simulink library "NCS_Library"  (R2019a)
settings: Solver=VariableStepAuto  StartTime=0.0  StopTime=10.0  RelTol=1e-3
values from neighbouring files (symbols this model uses):
  A = 10    [Parameter.m]
  band = 100000000    [Parameter.m]
  BER = 0    [Parameter.m]
  c = 5000000    [Parameter.m]
  c1 = 4.33    [Parameter.m]
  c2 = 3.16    [Parameter.m]
  CAN2EthernetDelay = 0.000    (= 0)    [Parameter.m]
  cR = 1.5*10^-3    (= 0.0015)    [Parameter.m]
  cw = (cwE * 2 + cwM * (nW_ges-2))/nW_ges    (= 0.1475)    [Parameter.m]
  cwE = 0.35    [Parameter.m]
  cwM = 0.08    [Parameter.m]
  Cycle_Controller = 0    [Parameter.m]
  CyclePLC = 24/1000    (= 0.024)    [Parameter.m]
  d = 800000    [Parameter.m]
  Dr = 0.92    [Parameter.m]
  Ethernet2CANDelay = 0.005    [Parameter.m]
  F_konst = 70892    [Parameter.m]
  FA = 100000    [Parameter.m]
  FB_WB_max = 10000    [Parameter.m]
  FBel_an = iG*nG*F_KZmax*nBan*R_mR/(Dr/2)    (= 28197.4297239)    [Parameter.m]
  FBel_frei = iG*nG*F_KZmax*nBfrei*R_mW/(Dr/2)    (= 29270.6882948)    [Parameter.m]
  Fmaxdyn = 300000    [Parameter.m]
  g = 9.81    [Parameter.m]
  i = 0    [Parameter.m]
  J = 1/2*mA*(Dr/2)^2    (= 158.7)    [Parameter.m]
  k1 = 0.095    [Parameter.m]
  k2 = 9.26/3.6    (= 2.57222222222)    [Parameter.m]
  k3 = 4.63/3.6    (= 1.28611111111)    [Parameter.m]
  mges = 58000    [Parameter.m]
  mu = [mu1 mu2]    [Parameter.m]
  muBel1 = 0.42    [Parameter.m]
  muBel2 = 0.36    [Parameter.m]
  n = 0.001    [Parameter.m]
  n_Mg = 4    [Parameter.m]
  n_WB = 4    [Parameter.m]
  nA = 4    [Parameter.m]
  nBan = 2    [Parameter.m]
  nBfrei = 3    [Parameter.m]
  nM = 4    [Parameter.m]
  nW_an = 4    [Parameter.m]
  P_max = 8200000    [Parameter.m]
  Q = 10    [Parameter.m]
  r_reib = 600    [Parameter.m]
  rho = 1.08    [Parameter.m]
  rhoL = 1.225    [Parameter.m]
  Size = 8    [Parameter.m]
  slip = [s1 s2]    [Parameter.m]
  tol = 0.05    [Parameter.m]
  v00 = 100/3.6    (= 27.7777777778)    [Parameter.m]
  v_grenz = 60/3.6    (= 16.6666666667)    [Parameter.m]
  v_opt = 75/3.6    (= 20.8333333333)    [Parameter.m]
  W_opt = 0.5    [Parameter.m]
  WB = 1    [Parameter.m]
  y_opt = sqrt(W_opt)/((1+sqrt(W_opt))^2+W_opt)    [Parameter.m]
undefined symbols (not defined in the file or in its folder): BUSCapacity, CableLength, controlGate, D_dyn, D_mg, EnableBurst, EnableToF, entity, Entity_out, Gate, Gate_4, Gate_5, Gate_ACK, Gate_copy, Gate_RX, getData, gettime, I_dyn, I_mg, m, magnitude, P_dyn, P_mg, ReadAttributes, readdata, ReadData, ReadSize, sigbuilder_block, Timeout, ToB, ToF, v0, v_d, v_soll
libraries: simulink x176, $bdroot x102
(part 7 of 12)

== system NCS_Library/Network/ETB/Subsystem2/MAC Layer ==
  InIP1 : Inport
  InFromIP2 : Inport  Port=2
  InFromIP3 : Inport  Port=3
  Parameter : Inport  Port=4
  InFromSubnet1 : Inport  Port=5
  InFromSubnet2 : Inport  Port=6
  InFromSubnet3 : Inport  Port=7
  Failure Control{,1..11} (12 alike) : $bdroot/Network/Applications/Failure Control  SystemSampleTime=-1
  MAC Controller1 : $bdroot/Network/ETB/OSI Layers/MAC Controller  SystemSampleTime=-1
  MAC Controller2 : $bdroot/Network/ETB/OSI Layers/MAC Controller  SystemSampleTime=-1
  MAC Controller3 : $bdroot/Network/ETB/OSI Layers/MAC Controller  SystemSampleTime=-1
  Terminator{,1..5} (6 alike) : Terminator
  OutIP1 : Outport
  OutToIP2 : Outport  Port=2
  OutToIP3 : Outport  Port=3
  OutToSubnet1 : Outport  Port=4
  OutSubnet2 : Outport  Port=5
  OutToSubnet3 : Outport  Port=6
  wires:
  MAC Controller1/1 -> Failure Control9/1
  MAC Controller1/4 -> Failure Control8/1
  InFromIP2/1 -> Failure Control7/1
  InFromSubnet2/1 -> Failure Control6/1
  MAC Controller2/4 -> Failure Control4/1
  MAC Controller2/1 -> Failure Control5/1
  InFromIP3/1 -> Failure Control1/1
  MAC Controller3/1 -> Failure Control3/1
  MAC Controller3/4 -> Failure Control2/1
  InFromSubnet3/1 -> Failure Control/1
  Parameter/1 -> MAC Controller3/2, MAC Controller2/2, MAC Controller1/2
  MAC Controller2/2 -> Terminator/1
  MAC Controller2/3 -> Terminator1/1
  MAC Controller3/2 -> Terminator2/1
  MAC Controller3/3 -> Terminator3/1
  MAC Controller1/3 -> Terminator4/1
  MAC Controller1/2 -> Terminator5/1
  InIP1/1 -> Failure Control11/1
  InFromSubnet1/1 -> Failure Control10/1
  Failure Control/1 -> MAC Controller3/3
  Failure Control1/1 -> MAC Controller3/1
  Failure Control2/1 -> OutToSubnet3/1
  Failure Control3/1 -> OutToIP3/1
  Failure Control4/1 -> OutSubnet2/1
  Failure Control5/1 -> OutToIP2/1
  Failure Control6/1 -> MAC Controller2/3
  Failure Control7/1 -> MAC Controller2/1
  Failure Control8/1 -> OutToSubnet1/1
  Failure Control9/1 -> OutIP1/1
  Failure Control10/1 -> MAC Controller1/3
  Failure Control11/1 -> MAC Controller1/1

== system NCS_Library/Network/ETB/Subsystem2/Routing Layer ==
  FIN : Inport
  Routing Table : Inport  Port=2
  Parameter : Inport  Port=3
  InSubnet3 : Inport  Port=4
  InSubnet2 : Inport  Port=5
  InSubnet1 : Inport  Port=6
  Display{1..6} (6 alike) : Display
  Entity Input Switch : EntityInputSwitch  InputPortMessageModes=m,m  OutputPortMessageModes=m
  Entity Input Switch1 : EntityInputSwitch  InputPortMessageModes=m,m  OutputPortMessageModes=m
  Entity Input Switch2 : EntityInputSwitch  InputPortMessageModes=m,m  OutputPortMessageModes=m
  Entity Output Switch1 : EntityOutputSwitch  InputPortMessageModes=m  OutputPortMessageModes=m,m  SwitchingCriterion=From attribute  SwitchAttributeName=CheckBit
  Entity Output Switch2 : EntityOutputSwitch  InputPortMessageModes=m  OutputPortMessageModes=m,m  SwitchingCriterion=From attribute  SwitchAttributeName=CheckBit
  Entity Output Switch3 : EntityOutputSwitch  InputPortMessageModes=m  OutputPortMessageModes=m,m  SwitchingCriterion=From attribute  SwitchAttributeName=CheckBit
  Entity Server1 : EntityServer  InputPortMessageModes=m  OutputPortMessageModes=n,m  Capacity=1  ServiceTimeValue=0  EntryAction=entity.CheckBit = entity.CheckBit+1;  NumberEntitiesDeparted=on
      settings: OutputPortMap=o0,o9
  Entity Server2 : EntityServer  InputPortMessageModes=m  OutputPortMessageModes=n,m  Capacity=1  ServiceTimeValue=0  EntryAction=entity.CheckBit = entity.CheckBit+1;  NumberEntitiesDeparted=on
      settings: OutputPortMap=o0,o9
  Entity Server3 : EntityServer  InputPortMessageModes=m  OutputPortMessageModes=n,m  Capacity=1  ServiceTimeValue=0  EntryAction=entity.CheckBit = entity.CheckBit+1;  NumberEntitiesDeparted=on
      settings: OutputPortMap=o0,o9
  Entity Terminator1 : EntityTerminator  InputPortMessageModes=m  NumberEntitiesArrived=on
      settings: OutputPortMap=o0
  Entity Terminator2 : EntityTerminator  InputPortMessageModes=m  NumberEntitiesArrived=on
      settings: OutputPortMap=o0
  Entity Terminator3 : EntityTerminator  InputPortMessageModes=m  NumberEntitiesArrived=on
      settings: OutputPortMap=o0
  FIN1 : InportShadow
  FIN2 : InportShadow
  Logic 1 : Subsystem
  Logic 2 : Subsystem
  Logic 3 : Subsystem
  Parameter4 : InportShadow  Port=3
  Parameter5 : InportShadow  Port=3
  Routing Table1 : InportShadow  Port=2
  Routing Table2 : InportShadow  Port=2
  OutSubnet3 : Outport
  OutSubnet2 : Outport  Port=2
  OutSubnet1 : Outport  Port=3
  wires:
  Entity Input Switch2/1 -> OutSubnet3/1
  Entity Input Switch1/1 -> OutSubnet1/1
  Entity Input Switch/1 -> OutSubnet2/1
  Entity Output Switch1/1 -> Entity Terminator1/1  "damaged"
  Entity Server1/2 -> Entity Output Switch1/1
  Entity Terminator1/1 -> Display3/1
  Entity Server1/1 -> Display1/1
  Routing Table2/1 -> Logic 3/2(Routing Table)
  Routing Table1/1 -> Logic 2/2(Routing Table)
  Parameter4/1 -> Logic 2/1(Parameter)
  Parameter5/1 -> Logic 3/1(Parameter)
  Parameter/1 -> Logic 1/1(Parameter)
  Routing Table/1 -> Logic 1/2(Routing Table)
  FIN/1 -> Logic 1/3(FIN_Init)
  Logic 1/1(Subnet 2) -> Entity Input Switch/1
  Entity Output Switch1/2 -> Logic 2/4(In)
  InSubnet2/1 -> Entity Server1/1
  FIN1/1 -> Logic 2/3(FIN_Init)
  Logic 3/2(Subnet 2) -> Entity Input Switch/2
  Logic 3/1(Subnet 1) -> Entity Input Switch1/2
  Logic 1/2(Subnet 3) -> Entity Input Switch2/1
  Logic 2/1(Subnet 1) -> Entity Input Switch1/1
  Logic 2/2(Subnet 3) -> Entity Input Switch2/2
  InSubnet3/1 -> Entity Server2/1
  Entity Output Switch2/1 -> Entity Terminator2/1  "damaged"
  Entity Server2/2 -> Entity Output Switch2/1
  Entity Server2/1 -> Display4/1
  Entity Terminator2/1 -> Display5/1
  Entity Output Switch2/2 -> Logic 3/4(In)
  InSubnet1/1 -> Entity Server3/1
  Entity Output Switch3/1 -> Entity Terminator3/1  "damaged"
  Entity Server3/2 -> Entity Output Switch3/1
  Entity Server3/1 -> Display2/1
  Entity Terminator3/1 -> Display6/1
  Entity Output Switch3/2 -> Logic 1/4(In)
  FIN2/1 -> Logic 3/3(FIN_Init)

== system NCS_Library/Network/ETB/Subsystem2/Routing Table ==
  Parameter : Inport
  Bus Selector : BusSelector  OutputSignals=RouterID,SubnetID1,SubnetID2,SubnetID3
  Get Routing Table : Subsystem
  Subsystem : Subsystem
  RT : Outport
  FIN : Outport  Port=2
  wires:
  Subsystem/1(Out1) -> Get Routing Table/5(Failed)
  Bus Selector/2 -> Get Routing Table/2(s1)  "<SubnetID1>"
  Parameter/1 -> Bus Selector/1
  Bus Selector/3 -> Get Routing Table/3(s2)  "<SubnetID2>"
  Bus Selector/1 -> Get Routing Table/1(RouterID)  "<RouterID>"
  Bus Selector/4 -> Get Routing Table/4(s3)  "<SubnetID3>"
  Get Routing Table/1(RT) -> RT/1
  Get Routing Table/2(FIN) -> FIN/1

== system NCS_Library/Network/ETB/Subsystem2/User Interface ==
  Bus Creator : BusCreator  Inputs=5
  Constant : Constant  Value=[ 0 0 ]  OutDataTypeStr=uint16
  Constant1 : Constant  Value=0  OutDataTypeStr=uint16
  Data Type Conversion : DataTypeConversion  OutDataTypeStr=uint16
  Mux : Mux  Inputs=3
  RouterID : Constant  Value=RouterID  OutMin=1  OutMax=99  OutDataTypeStr=uint8
  connected SubNetID 1 : Constant  Value=SubnetIDa  OutMin=0  OutMax=399  OutDataTypeStr=uint16
  connected SubNetID 2 : Constant  Value=SubnetIDb  OutMin=0  OutMax=399  OutDataTypeStr=uint16
  connected SubNetID 3 : Constant  Value=SubnetIDc  OutMin=0  OutMax=399  OutDataTypeStr=uint16
  Paramter : Outport
  wires:
  RouterID/1 -> Bus Creator/5, Data Type Conversion/1  "RouterID"
  connected SubNetID 3/1 -> Bus Creator/3  "SubnetID3"
  connected SubNetID 2/1 -> Bus Creator/2  "SubnetID2"
  connected SubNetID 1/1 -> Bus Creator/1  "SubnetID1"
  Mux/1 -> Bus Creator/4  "Address"
  Bus Creator/1 -> Paramter/1
  Constant/1 -> Mux/3
  Data Type Conversion/1 -> Mux/2
  Constant1/1 -> Mux/1

== system NCS_Library/Network/Gateway/Gateway1/CAN Interface ==
  ReceivedData : Inport
  Buffer Overflow : EntityTerminator  InputPortMessageModes=m  NumberEntitiesArrived=on
      settings: OutputPortMap=o0
  CAN Interface : Subsystem
  Display{2..4,9} (4 alike) : Display
  Entity Output Switch : EntityOutputSwitch  InputPortMessageModes=m  OutputPortMessageModes=m,m  SwitchAttributeName=Attribute1
  Entity Gate2 : EntityGate  InputPortMessageModes=m,m  OutputPortMessageModes=m
  Entity Gate3 : EntityGate  InputPortMessageModes=m,m  OutputPortMessageModes=m  OperatingMode=Release gate
  Entity Terminator1 : EntityTerminator  InputPortMessageModes=m  NumberEntitiesArrived=on
      settings: OutputPortMap=o0
  Entry Control : Subsystem
  Gate Control : Subsystem
  Message Send1 : MessageSend  OutputPortMessageModes=m
      settings: InputPortMap=u1
  Multicast Receive Queue : EntityQueue  InputPortMessageModes=m  OutputPortMessageModes=n,m  Capacity=100  EntryAction=ReadData(entity.SensorType,entity.Data);  NumberEntitiesInBlock=on
      settings: OutputPortMap=o1,o5
  Multicast Receive Queue1 : EntityQueue  InputPortMessageModes=m  OutputPortMessageModes=n,m  Capacity=inf  NumberEntitiesInBlock=on
      settings: OutputPortMap=o1,o5
  Read Data : Subsystem  TreatAsAtomicUnit=on
  Save Data : Subsystem
  Transport Delay : TransportDelay  DelayTime=CAN2EthernetDelay
  OutEthernetData : Outport
  wires:
  Gate Control/1(FLUSH) -> Save Data/3(FLUSH), Entry Control/1(FLUSH), Message Send1/1
  Read Data/1(Type) -> Save Data/1(Type)
  CAN Interface/1(CAN_Message) -> Entity Output Switch/1
  Read Data/2(Data) -> Save Data/2(Data)
  Entity Terminator1/1 -> Display3/1
  Entity Output Switch/1 -> Multicast Receive Queue1/1
  Buffer Overflow/1 -> Display2/1
  Entity Output Switch/2 -> Buffer Overflow/1
  Multicast Receive Queue/1 -> Display4/1, Entry Control/2(n_packets), Gate Control/1(n_packets)
  Multicast Receive Queue/2 -> Entity Gate2/2
  Multicast Receive Queue1/1 -> Display9/1
  Entry Control/1(Out1) -> Entity Gate3/1
  Message Send1/1 -> Entity Gate2/1
  Multicast Receive Queue1/2 -> Entity Gate3/2
  Entity Gate3/1 -> Multicast Receive Queue/1
  Entity Gate2/1 -> Entity Terminator1/1
  Save Data/1(OutData) -> Transport Delay/1
  ReceivedData/1 -> CAN Interface/1(d_in)
  Transport Delay/1 -> OutEthernetData/1

== system NCS_Library/Network/Gateway/Gateway1/Ethernet Interface ==
  RxFromBus : Inport
  CANData : Inport  Port=2
  Buffer : MATLAB Function  TreatAsAtomicUnit=on
  Display : Display
  Display1 : Display
  Display2 : Display
  Enabled Subsystem : Subsystem  TreatAsAtomicUnit=on
  Failure Control : $bdroot/Network/Applications/Failure Control  SystemSampleTime=-1
  Failure Control1 : $bdroot/Network/Applications/Failure Control  SystemSampleTime=-1
  Memory : Memory  InitialCondition=zeros(3,100)  InheritSampleTime=on
  Protocol Stack : Subsystem
  Subsystem4 : Subsystem
  Terminator : Terminator
  Transport Delay : TransportDelay  DelayTime=Ethernet2CANDelay
  User Interface : Subsystem
  TxToBus : Outport
  ReceivedData : Outport  Port=2
  wires:
  CANData/1 -> Protocol Stack/1(Signal)
  Failure Control/1 -> Protocol Stack/3(RxFromBus)
  Failure Control1/1 -> TxToBus/1
  RxFromBus/1 -> Failure Control/1
  Protocol Stack/3(TxToBus) -> Failure Control1/1
  Protocol Stack/2(Recorder) -> Terminator/1
  Buffer/1(Buffer) -> Memory/1, Display/1
  Memory/1 -> Buffer/1(updatedBuffer)
  Protocol Stack/1(Data) -> Transport Delay/1
  Subsystem4/1(Push) -> Display2/1, Enabled Subsystem/Enable, Buffer/2(Push)
  Buffer/2(data) -> Enabled Subsystem/1(In1)
  Enabled Subsystem/1(Out1) -> Display1/1, ReceivedData/1
  Transport Delay/1 -> Subsystem4/1(Data), Buffer/3(Data)
  User Interface/1(Out1) -> Protocol Stack/2(Parameter)

== system NCS_Library/Network/Gateway/Gateway2/CAN Interface ==
  ReceivedData : Inport
  Buffer Overflow : EntityTerminator  InputPortMessageModes=m  NumberEntitiesArrived=on
      settings: OutputPortMap=o0
  CAN Interface : Subsystem
  Display{2..4,9} (4 alike) : Display
  Entity Output Switch : EntityOutputSwitch  InputPortMessageModes=m  OutputPortMessageModes=m,m  SwitchAttributeName=Attribute1
  Entity Gate2 : EntityGate  InputPortMessageModes=m,m  OutputPortMessageModes=m
  Entity Gate3 : EntityGate  InputPortMessageModes=m,m  OutputPortMessageModes=m  OperatingMode=Release gate
  Entity Terminator1 : EntityTerminator  InputPortMessageModes=m  NumberEntitiesArrived=on
      settings: OutputPortMap=o0
  Entry Control : Subsystem
  Gate Control : Subsystem
  Message Send1 : MessageSend  OutputPortMessageModes=m
      settings: InputPortMap=u1
  Multicast Receive Queue : EntityQueue  InputPortMessageModes=m  OutputPortMessageModes=n,m  Capacity=100  EntryAction=ReadData(entity.SensorType,entity.Data);  NumberEntitiesInBlock=on
      settings: OutputPortMap=o1,o5
  Multicast Receive Queue1 : EntityQueue  InputPortMessageModes=m  OutputPortMessageModes=n,m  Capacity=inf  NumberEntitiesInBlock=on
      settings: OutputPortMap=o1,o5
  Read Data : Subsystem  TreatAsAtomicUnit=on
  Save Data : Subsystem
  Transport Delay : TransportDelay  DelayTime=CAN2EthernetDelay
  OutEthernetData : Outport
  wires:
  Transport Delay/1 -> OutEthernetData/1
  ReceivedData/1 -> CAN Interface/1(d_in)
  Save Data/1(OutData) -> Transport Delay/1
  Entity Gate2/1 -> Entity Terminator1/1
  Entity Gate3/1 -> Multicast Receive Queue/1
  Multicast Receive Queue1/2 -> Entity Gate3/2
  Message Send1/1 -> Entity Gate2/1
  Entry Control/1(Out1) -> Entity Gate3/1
  Multicast Receive Queue1/1 -> Display9/1
  Multicast Receive Queue/2 -> Entity Gate2/2
  Multicast Receive Queue/1 -> Gate Control/1(n_packets), Entry Control/2(n_packets), Display4/1
  Entity Output Switch/2 -> Buffer Overflow/1
  Buffer Overflow/1 -> Display2/1
  Entity Output Switch/1 -> Multicast Receive Queue1/1
  Entity Terminator1/1 -> Display3/1
  Read Data/2(Data) -> Save Data/2(Data)
  CAN Interface/1(CAN_Message) -> Entity Output Switch/1
  Read Data/1(Type) -> Save Data/1(Type)
  Gate Control/1(FLUSH) -> Message Send1/1, Entry Control/1(FLUSH), Save Data/3(FLUSH)

== system NCS_Library/Network/Gateway/Gateway2/Ethernet Interface ==
  note: User defined Parameters
  RxFromBus : Inport
  CANData : Inport  Port=2
  Add : Sum  Inputs=+-
  Buffer : MATLAB Function  TreatAsAtomicUnit=on
  Bus Creator : BusCreator  Inputs=8
  Constant : Constant  Value=Address  OutDataTypeStr=uint16
  Constant1 : Constant  Value=Destination  OutDataTypeStr=uint16
  Constant2 : Constant  Value=0  OutDataTypeStr=double
  Constant3 : Constant  Value=3  OutDataTypeStr=uint8
  Constant4 : Constant  Value=SDTv2  OutDataTypeStr=double
  Constant5 : Constant
  Constant6 : Constant  Value=Port  OutDataTypeStr=uint16
  Constant7 : Constant  Value=ReplyAddress  OutDataTypeStr=uint16
  Display : Display
  Display1 : Display
  Display2 : Display
  Enabled Subsystem : Subsystem  TreatAsAtomicUnit=on
  Failure Control : $bdroot/Network/Applications/Failure Control  SystemSampleTime=-1
  Failure Control1 : $bdroot/Network/Applications/Failure Control  SystemSampleTime=-1
  MATLAB Function : MATLAB Function  TreatAsAtomicUnit=on
  MATLAB Function1 : MATLAB Function  TreatAsAtomicUnit=on
  Memory : Memory  InitialCondition=zeros(3,100)  InheritSampleTime=on
  Subscribe : Constant  Value=Subscribe  OutDataTypeStr=uint16
  Subsystem : Subsystem
  Subsystem1 : Subsystem
  Subsystem2 : Subsystem
  Subsystem3 : Subsystem
  Subsystem4 : Subsystem
  Terminator : Terminator
  Transport Delay : TransportDelay  DelayTime=Ethernet2CANDelay
  TxToBus : Outport
  ReceivedData : Outport  Port=2
  wires:
  Transport Delay/1 -> Buffer/3(Data), Subsystem4/1(Data)
  Enabled Subsystem/1(Out1) -> ReceivedData/1, Display1/1
  Buffer/2(data) -> Enabled Subsystem/1(In1)
  Subsystem4/1(Push) -> Buffer/2(Push), Enabled Subsystem/Enable, Display2/1
  Subsystem/1(Data) -> Transport Delay/1
  Memory/1 -> Buffer/1(updatedBuffer)
  Buffer/1(Buffer) -> Memory/1, Display/1
  Subsystem/2(Recorder) -> Terminator/1
  Constant5/1 -> Add/2
  MATLAB Function/1(msgType) -> Bus Creator/7  "msgType"
  Constant1/1 -> Subsystem2/1(In1)
  Subsystem/3(TxToBus) -> Failure Control1/1
  RxFromBus/1 -> Failure Control/1
  Failure Control1/1 -> TxToBus/1
  Constant6/1 -> Bus Creator/5  "Port"
  Bus Creator/1 -> Subsystem/2(Parameter)
  Failure Control/1 -> Subsystem/3(RxFromBus)
  CANData/1 -> Subsystem/1(Signal)
  MATLAB Function1/1(y) -> Bus Creator/3  "Subscribe"
  Constant2/1 -> Bus Creator/6  "T_Tx"
  Constant7/1 -> Subsystem3/1(In1)
  Subsystem3/1(Out1) -> Bus Creator/4  "ReplyAddress"
  Subscribe/1 -> MATLAB Function1/1(u)
  Constant3/1 -> MATLAB Function/1(u)
  Subsystem1/1(Out1) -> Bus Creator/1  "Address"
  Constant/1 -> Subsystem1/1(In1)
  Constant4/1 -> Add/1
  Subsystem2/1(Out1) -> Bus Creator/2  "Destination"
  Add/1 -> Bus Creator/8  "SDTv2"

== system NCS_Library/Plant (Train)/Angetriebene_Achse/Bremskraft pro angetriebener Achse2/Belagreibwert_Nennwerte ==
  v : Inport
  Add : Sum
  Add1 : Sum
  Compare To Constant : simulink/Logic and Bit Operations/Compare To Constant  relop=<=  const=200/3.6  OutDataTypeStr=boolean
  Compare To Constant3 : simulink/Logic and Bit Operations/Compare To Constant  relop=>  const=200/3.6  OutDataTypeStr=boolean
  Compare To Constant4 : simulink/Logic and Bit Operations/Compare To Constant  relop=>=  const=0  OutDataTypeStr=boolean
  Constant1 : Constant  Value=muBel1
  Constant6 : Constant  Value=muBel1-muBel2
  Gain1 : Gain  Gain=3.6/100
  Gain2 : Gain  Gain=2
  Product1 : Product  Inputs=3
  Product3 : Product
  Product4 : Product
  Subtract1 : Sum  Inputs=+-
  mu_Bel : Outport
  wires:
  Compare To Constant/1 -> Product1/3
  Constant1/1 -> Add1/1, Product1/2
  Compare To Constant3/1 -> Product3/1
  v/1 -> Compare To Constant4/1, Product4/2, Compare To Constant3/1, Compare To Constant/1
  Add1/1 -> Subtract1/1
  Constant6/1 -> Gain2/1, Gain1/1
  Gain1/1 -> Product4/1
  Product4/1 -> Subtract1/2
  Subtract1/1 -> Product3/2
  Product1/1 -> Add/1
  Product3/1 -> Add/2
  Add/1 -> mu_Bel/1
  Compare To Constant4/1 -> Product1/1
  Gain2/1 -> Add1/2

== system NCS_Library/Plant (Train)/Angetriebene_Achse/Bremskraft pro angetriebener Achse2/max dynamische Bremse pro angetriebener Achse1 ==
  v : Inport
  Add2 : Sum  Inputs=+++
  Add3 : Sum
  Compare To Constant4 : simulink/Logic and Bit Operations/Compare To Constant  relop=<=  const=29  OutDataTypeStr=boolean
  Compare To Constant5 : simulink/Logic and Bit Operations/Compare To Constant  relop=>  const=29  OutDataTypeStr=boolean
  Compare To Constant6 : simulink/Logic and Bit Operations/Compare To Constant  relop=>  const=4.2  OutDataTypeStr=boolean
  Compare To Constant7 : simulink/Logic and Bit Operations/Compare To Constant  relop=<=  const=4.2  OutDataTypeStr=boolean
  Compensate v=0 : Constant  Value=1e-10
  Display : Display
  Fmax2 : Constant  Value=Fmaxdyn
  Fmax3 : Constant  Value=F_konst
  Gain1 : Gain  Gain=1/(nA*nW_an)
  Gain2 : Gain  Gain=r_reib
  Leistung1 : Constant  Value=P_max
  Logical Operator1 : Logic  AllPortsSameDT=off  OutDataTypeStr=boolean
  Product3 : Product
  Product4 : Product  Inputs=*/*
  Product5 : Product  Inputs=3
  Subtract1 : Sum  Inputs=+-
  F_B,dyn_max : Outport
  wires:
  Gain1/1 -> F_B,dyn_max/1
  Product4/1 -> Add2/3
  v/1 -> Compare To Constant7/1, Product5/3, Compare To Constant6/1, Compare To Constant4/1, Gain2/1, Add3/1, Compare To Constant5/1
  Compare To Constant5/1 -> Product4/3
  Subtract1/1 -> Product3/1
  Fmax2/1 -> Subtract1/1
  Add2/1 -> Gain1/1
  Compare To Constant7/1 -> Product5/2
  Fmax3/1 -> Product5/1
  Product3/1 -> Add2/2, Display/1
  Product5/1 -> Add2/1
  Add3/1 -> Product4/2
  Leistung1/1 -> Product4/1
  Logical Operator1/1 -> Product3/2
  Compare To Constant6/1 -> Logical Operator1/2
  Gain2/1 -> Subtract1/2
  Compensate v=0/1 -> Add3/2
  Compare To Constant4/1 -> Logical Operator1/1

== system NCS_Library/Plant (Train)/Angetriebene_Achse/Bremskraft pro angetriebener Achse2/max dynamische Motor pro angetriebener Achse ==
  v : Inport
  Add2 : Sum
  Add3 : Sum
  Compare To Constant4 : simulink/Logic and Bit Operations/Compare To Constant  relop=<=  const=29  OutDataTypeStr=boolean
  Compare To Constant5 : simulink/Logic and Bit Operations/Compare To Constant  relop=>  const=29  OutDataTypeStr=boolean
  Compensate v=0 : Constant  Value=1e-10
  Display : Display
  Display1 : Display
  Display2 : Display
  Fmax2 : Constant  Value=Fmaxdyn
  Gain1 : Gain  Gain=1/(nA*nW_an)
  Gain2 : Gain  Gain=r_reib
  Leistung1 : Constant  Value=P_max
  Product3 : Product
  Product4 : Product  Inputs=*/*
  Subtract1 : Sum  Inputs=+-
  F_B,dyn_max : Outport
  wires:
  Compensate v=0/1 -> Add3/2
  Gain2/1 -> Subtract1/2
  Compare To Constant4/1 -> Product3/2
  Leistung1/1 -> Product4/1
  Add3/1 -> Product4/2
  Product3/1 -> Display/1, Add2/1
  Add2/1 -> Gain1/1
  Fmax2/1 -> Subtract1/1
  Subtract1/1 -> Product3/1
  Compare To Constant5/1 -> Product4/3
  Product4/1 -> Display1/1, Add2/2
  Gain1/1 -> F_B,dyn_max/1
  v/1 -> Display2/1, Compare To Constant5/1, Add3/1, Gain2/1, Compare To Constant4/1

== system NCS_Library/Plant (Train)/Freie_Achse/Bremskraft pro freier Achse1/Belagreibwert_Nennwerte ==
  v : Inport
  Add : Sum
  Add1 : Sum
  Compare To Constant : simulink/Logic and Bit Operations/Compare To Constant  relop=<=  const=200/3.6  OutDataTypeStr=boolean
  Compare To Constant3 : simulink/Logic and Bit Operations/Compare To Constant  relop=>  const=200/3.6  OutDataTypeStr=boolean
  Compare To Constant4 : simulink/Logic and Bit Operations/Compare To Constant  relop=>=  const=0  OutDataTypeStr=boolean
  Constant1 : Constant  Value=muBel1
  Constant6 : Constant  Value=muBel1-muBel2
  Gain1 : Gain  Gain=3.6/100
  Gain2 : Gain  Gain=2
  Product1 : Product  Inputs=3
  Product3 : Product
  Product4 : Product
  Subtract1 : Sum  Inputs=+-
  muBel : Outport
  wires:
  Gain2/1 -> Add1/2
  Compare To Constant4/1 -> Product1/1
  Add/1 -> muBel/1
  Product3/1 -> Add/2
  Product1/1 -> Add/1
  Subtract1/1 -> Product3/2
  Product4/1 -> Subtract1/2
  Gain1/1 -> Product4/1
  Constant6/1 -> Gain1/1, Gain2/1
  Add1/1 -> Subtract1/1
  v/1 -> Compare To Constant/1, Compare To Constant3/1, Product4/2, Compare To Constant4/1
  Compare To Constant3/1 -> Product3/1
  Constant1/1 -> Product1/2, Add1/1
  Compare To Constant/1 -> Product1/3

== system NCS_Library/Plant (Train)/angetriebener Endwagen Merz/Achse_1/Bremskraft pro angetriebener Achse1 ==
  v : Inport
  fSt_dyn : Inport  Port=2
  Bremsstufenfaktor A1 : Inport  Port=3
  Add : Sum
  Belagreibwert_Nennwerte : Subsystem
  Belagskraft pro Achse : Constant  Value=FBel_an
  Compare To Constant3 : simulink/Logic and Bit Operations/Compare To Constant  relop=>=  const=0  OutDataTypeStr=boolean
  Product : Product  Inputs=3
  Product1 : Product  Inputs=3
  anliegende Bremskraft : Scope
  dynamische Bremskraft : Scope
  max dynamische Bremse pro angetriebener Achse : Subsystem
  müh : Scope
  pneumatik Bremse Bremskraft : Scope
  FBA : Outport
  wires:
  Belagskraft pro Achse/1 -> Product/2
  Bremsstufenfaktor A1/1 -> Product/3
  v/1 -> Belagreibwert_Nennwerte/1(v), max dynamische Bremse pro angetriebener Achse/1(v), Compare To Constant3/1
  Belagreibwert_Nennwerte/1(mühBel) -> müh/1, Product/1
  Product/1 -> pneumatik Bremse Bremskraft/1, Add/2
  Add/1 -> FBA/1, anliegende Bremskraft/1
  Product1/1 -> Add/1, dynamische Bremskraft/1
  max dynamische Bremse pro angetriebener Achse/1(FB) -> Product1/2
  Compare To Constant3/1 -> Product1/3
  fSt_dyn/1 -> Product1/1

== system NCS_Library/Plant (Train)/angetriebener Endwagen Merz/Achse_2/Bremskraft pro angetriebener Achse2 ==
  v : Inport
  fSt_dyn : Inport  Port=2
  Bremsstufenfaktor A2 : Inport  Port=3
  Add : Sum
  Belagreibwert_Nennwerte : Subsystem
  Belagskraft pro Achse : Constant  Value=FBel_an
  Compare To Constant3 : simulink/Logic and Bit Operations/Compare To Constant  relop=>=  const=0  OutDataTypeStr=boolean
  Product : Product  Inputs=3
  Product1 : Product  Inputs=3
  max dynamische Bremse pro angetriebener Achse : Subsystem
  FBA : Outport
  wires:
  Belagreibwert_Nennwerte/1(mühBel) -> Product/1
  Belagskraft pro Achse/1 -> Product/2
  Bremsstufenfaktor A2/1 -> Product/3
  v/1 -> Belagreibwert_Nennwerte/1(v), Compare To Constant3/1, max dynamische Bremse pro angetriebener Achse/1(v)
  Product/1 -> Add/2
  Add/1 -> FBA/1
  Product1/1 -> Add/1
  max dynamische Bremse pro angetriebener Achse/1(FB) -> Product1/2
  Compare To Constant3/1 -> Product1/3
  fSt_dyn/1 -> Product1/1

== system NCS_Library/Plant (Train)/angetriebener Endwagen Merz/Achse_3/Bremskraft pro angetriebener Achse3 ==
  v : Inport
  fSt_dyn : Inport  Port=2
  Bremsstufenfaktor A3 : Inport  Port=3
  Add : Sum
  Belagreibwert_Nennwerte : Subsystem
  Belagskraft pro Achse : Constant  Value=FBel_an
  Compare To Constant3 : simulink/Logic and Bit Operations/Compare To Constant  relop=>=  const=0  OutDataTypeStr=boolean
  Product : Product  Inputs=3
  Product1 : Product  Inputs=3
  max dynamische Bremse pro angetriebener Achse : Subsystem
  FBA : Outport
  wires:
  Belagskraft pro Achse/1 -> Product/2
  Bremsstufenfaktor A3/1 -> Product/3
  v/1 -> Belagreibwert_Nennwerte/1(v), Compare To Constant3/1, max dynamische Bremse pro angetriebener Achse/1(v)
  Belagreibwert_Nennwerte/1(mühBel) -> Product/1
  Product/1 -> Add/2
  Add/1 -> FBA/1
  Product1/1 -> Add/1
  max dynamische Bremse pro angetriebener Achse/1(FB) -> Product1/2
  Compare To Constant3/1 -> Product1/3
  fSt_dyn/1 -> Product1/1

== system NCS_Library/Plant (Train)/angetriebener Endwagen Merz/Achse_4/Bremskraft pro angetriebener Achse4 ==
  v : Inport
  fSt_dyn : Inport  Port=2
  Bremsstufenfaktor A4 : Inport  Port=3
  Add : Sum
  Belagreibwert_Nennwerte : Subsystem
  Belagskraft pro Achse : Constant  Value=FBel_an
  Compare To Constant3 : simulink/Logic and Bit Operations/Compare To Constant  relop=>=  const=0  OutDataTypeStr=boolean
  Product : Product  Inputs=3
  Product1 : Product  Inputs=3
  max dynamische Bremse pro angetriebener Achse : Subsystem
  FBA : Outport
  wires:
  Belagskraft pro Achse/1 -> Product/2
  Bremsstufenfaktor A4/1 -> Product/3
  v/1 -> Belagreibwert_Nennwerte/1(v), Compare To Constant3/1, max dynamische Bremse pro angetriebener Achse/1(v)
  Belagreibwert_Nennwerte/1(mühBel) -> Product/1
  Product/1 -> Add/2
  Add/1 -> FBA/1
  Product1/1 -> Add/1
  max dynamische Bremse pro angetriebener Achse/1(FB) -> Product1/2
  Compare To Constant3/1 -> Product1/3
  fSt_dyn/1 -> Product1/1

== system NCS_Library/Plant (Train)/angetriebener Endwagen Merz/Wagen/Fahrwiderstand_Wagen ==
  note: Widerstand durch Kühlung der Bremsscheiben
  note: Luftwiderstand
  note: Motorkühlung und Klimatisierung
  note: Rollwiderstand
  note: Streckenwiderstand
  v : Inport
  Neigung in Promille : Inport  Port=2
  mges : Inport  Port=3
  Achsenanzahl : Constant  Value=nA
  Add : Sum  Inputs=+++++
  Add1 : Sum
  Anorm : Constant  Value=A
  Bremsscheibenanzahl : Constant  Value=nBan
  Compare To Zero : simulink/Logic and Bit Operations/Compare To Zero  relop=>  OutDataTypeStr=boolean
  Divide1 : Product  Inputs=*/
  Gain : Gain  Gain=1/1000
  Gain1 : Gain  Gain=1/2
  Luftdurchsatz : Constant  Value=Q
  Math Function : Math  Operator=magnitude^2  SaturateOnIntegerOverflow=on
  Math Function1 : Math  Operator=magnitude^2  SaturateOnIntegerOverflow=on
  Product : Product  Inputs=3
  Product1 : Product  Inputs=4
  Product2 : Product  Inputs=4
  Product{3..5,7..8} (5 alike) : Product
  Product6 : Product  Inputs=3
  Trigonometric Function : Trigonometry  Operator=atan
  Trigonometric Function1 : Trigonometry
  Trigonometric Function2 : Trigonometry  Operator=cos
  c1 : Constant  Value=c1
  c2 : Constant  Value=c2
  cR : Constant  Value=cR
  cw : Constant  Value=cwE
  g : Constant  Value=g
  g1 : Constant  Value=g
  rhoLuft : Constant  Value=rhoL
  v00 : Constant  Value=v00
  Fw : Outport
  wires:
  Trigonometric Function2/1 -> Product1/4
  Bremsscheibenanzahl/1 -> Product8/2
  Product8/1 -> Product3/1
  Compare To Zero/1 -> Product7/1
  Product7/1 -> Fw/1
  Math Function1/1 -> Product5/2
  Product6/1 -> Add/3
  Luftdurchsatz/1 -> Product6/3
  c2/1 -> Product5/1
  Math Function/1 -> Product2/1
  Divide1/1 -> Math Function1/1, Product4/2
  Product5/1 -> Add1/2
  Product4/1 -> Add1/1
  v00/1 -> Divide1/2
  c1/1 -> Product4/1
  Add1/1 -> Product3/2
  Product3/1 -> Add/1
  Achsenanzahl/1 -> Product8/1
  Product2/1 -> Add/2
  Gain1/1 -> Product2/4
  cw/1 -> Product2/3
  Anorm/1 -> Product2/2
  v/1 -> Math Function/1, Divide1/1, Compare To Zero/1, Product6/2
  rhoLuft/1 -> Gain1/1, Product6/1
  Product1/1 -> Add/4
  mges/1 -> Product1/3, Product/2
  cR/1 -> Product1/2
  g1/1 -> Product1/1
  Add/1 -> Product7/2
  Product/1 -> Add/5
  Trigonometric Function1/1 -> Product/3
  g/1 -> Product/1
  Gain/1 -> Trigonometric Function/1
  Trigonometric Function/1 -> Trigonometric Function1/1, Trigonometric Function2/1
  Neigung in Promille/1 -> Gain/1

== system NCS_Library/Plant (Train)/freier Wagen/Bremskraft Schienenbremse/Mg-Bremse pro Wagen ==
  v : Inport
  Add : Sum
  Add1 : Sum
  Constant : Constant  Value=FA
  Constant1 : Constant  Value=k1
  Constant2 : Constant  Value=k2
  Constant3 : Constant  Value=k3
  Constant4 : Constant  Value=n_Mg
  Divide : Product  Inputs=*/
  Product : Product  Inputs=4
  Out1 : Outport
  wires:
  Constant1/1 -> Product/2
  Constant2/1 -> Add/1
  Constant3/1 -> Add1/2
  Add/1 -> Divide/1
  Add1/1 -> Divide/2
  Divide/1 -> Product/3
  Constant/1 -> Product/4
  Product/1 -> Out1/1
  Constant4/1 -> Product/1
  v/1 -> Add1/1, Add/2

== system NCS_Library/Plant (Train)/freier Wagen/Bremskraft Schienenbremse/WB Bremse pro Wagen ==
  v : Inport
  Constant : Constant  Value=FB_WB_max
  Constant2 : Constant  Value=y_opt
  Divide : Product  Inputs=*/
  Gain : Gain  Gain=n_WB
  Product : Product
  Subsystem : Subsystem
  Fb_WB : Outport
  wires:
  Product/1 -> Divide/1
  Subsystem/1(y) -> Product/1
  Constant/1 -> Product/2
  Constant2/1 -> Divide/2
  Divide/1 -> Gain/1
  Gain/1 -> Fb_WB/1
  v/1 -> Subsystem/1(v)

== system NCS_Library/Controller/Logic/Braking Controller/konstante Fahrt/Fahrwiderstand ==
  note: warum addition ??
  v : Inport
  Add : Sum
  Fahrwiderstand_angeWagen : Subsystem
  Fahrwiderstand_freiWagen : Subsystem
  F_W : Outport
  wires:
  Add/1 -> F_W/1
  v/1 -> Fahrwiderstand_angeWagen/1(v), Fahrwiderstand_freiWagen/1(v)
  Fahrwiderstand_freiWagen/1(F_W) -> Add/2
  Fahrwiderstand_angeWagen/1(F_W) -> Add/1

== system NCS_Library/Controller/Logic/Braking Controller/konstante Fahrt/Subsystem ==
  FW : Inport
  FB : Inport  Port=2
  Add : Sum
  Compare To Zero : simulink/Logic and Bit Operations/Compare To Zero  relop=<  OutDataTypeStr=boolean
  Compare To Zero1 : simulink/Logic and Bit Operations/Compare To Zero  relop=>=  OutDataTypeStr=boolean
  Constant : Constant  Value=0
  Divide : Product  Inputs=*/
  Divide2 : Product  Inputs=*/
  FB1 : InportShadow  Port=2
  FB2 : InportShadow  Port=2
  FW1 : InportShadow
  FW2 : InportShadow
  Gain : Gain  Gain=-1
  Gain1 : Gain  Gain=nW_an/nM
  Gain2 : Gain  Gain=-1
  Product : Product
  Product1 : Product
  Saturation : Saturate  UpperLimit=1  LowerLimit=0
  Switch : Switch  Criteria=u2 > Threshold
  Motor : Outport
  wires:
  Product/1 -> Gain1/1  "F_B"
  Product1/1 -> Gain2/1  "fSt_dyn"
  Gain/1 -> Divide2/2
  Gain1/1 -> Add/1
  FW/1 -> Compare To Zero1/1, Divide2/1
  Saturation/1 -> Add/2  "fSt_dyn"
  FB/1 -> Gain/1
  Divide/1 -> Product1/2
  Compare To Zero/1 -> Product1/1
  Gain2/1 -> Saturation/1
  Compare To Zero1/1 -> Product/1
  Add/1 -> Switch/1  "Motor"
  FW1/1 -> Compare To Zero/1
  FW2/1 -> Divide/1
  FB1/1 -> Divide/2
  Divide2/1 -> Product/2
  Switch/1 -> Motor/1
  FB2/1 -> Switch/2
  Constant/1 -> Switch/3

== system NCS_Library/Controller/Logic/Braking Controller/konstante Fahrt/Subsystem1 ==
  F_W : Inport
  F_B,dyn_max : Inport  Port=2
  F_B,WB : Inport  Port=3
  v : Inport  Port=4
  Add : Sum  Inputs=+|-||
  Compare To Constant1 : simulink/Logic and Bit Operations/Compare To Constant  relop=>  const=v_grenz  OutDataTypeStr=boolean
  Compare To Constant7 : simulink/Logic and Bit Operations/Compare To Constant  relop=>  const=0  OutDataTypeStr=boolean
  Compare To Zero2 : simulink/Logic and Bit Operations/Compare To Zero  relop=<  OutDataTypeStr=boolean
  Constant : Constant  Value=0
  Constant1 : Constant  Value=2
  Constant10 : Constant  Value=WB
  Divide1 : Product  Inputs=*/
  Gain3 : Gain  Gain=-1
  Multiport Switch : MultiPortSwitch  Inputs=2
  Product2 : Product
  Product6 : Product
  Subtract : Sum
  Schienenbremse : Outport
  wires:
  Compare To Zero2/1 -> Product2/1
  Constant10/1 -> Compare To Constant7/1
  Gain3/1 -> Product6/1
  F_B,dyn_max/1 -> Subtract/2
  Subtract/1 -> Divide1/1, Compare To Zero2/1
  Compare To Constant7/1 -> Product6/2
  Divide1/1 -> Product2/2
  F_B,WB/1 -> Divide1/2
  Product2/1 -> Gain3/1  "f_St,WB"
  F_W/1 -> Subtract/1
  Product6/1 -> Multiport Switch/2  "Schienenbremse"
  v/1 -> Compare To Constant1/1
  Multiport Switch/1 -> Schienenbremse/1
  Constant/1 -> Multiport Switch/3
  Add/1 -> Multiport Switch/1
  Compare To Constant1/1 -> Add/2
  Constant1/1 -> Add/1

== system NCS_Library/Controller/Logic/Braking Controller/konstante Fahrt/WB Bremse pro Wagen ==
  v : Inport
  Add : Sum
  Bremse abschalten : simulink/Logic and Bit Operations/Compare To Constant  relop=>  const=v_grenz+5/3.6  OutDataTypeStr=boolean
  Compare To Constant : simulink/Logic and Bit Operations/Compare To Constant  relop=<=  const=v_grenz+5/3.6  OutDataTypeStr=boolean
  Compare To Constant1 : simulink/Logic and Bit Operations/Compare To Constant  relop=>  const=v_grenz  OutDataTypeStr=boolean
  Constant : Constant  Value=FB_WB_max
  Constant1 : Constant  Value=v_grenz
  Constant2 : Constant  Value=y_opt
  Gain : Gain  Gain=n_WB
  Gain1 : Gain  Gain=0.72
  Logical Operator : Logic  AllPortsSameDT=off  OutDataTypeStr=boolean
  Product : Product  Inputs=***/
  Product1 : Product
  Subsystem : Subsystem
  Subtract : Sum  Inputs=-+
  F_B,WB : Outport
  wires:
  Logical Operator/1 -> Gain1/1
  Gain1/1 -> Product1/2
  Compare To Constant1/1 -> Logical Operator/2
  Add/1 -> Product/1  "f_St,WB ?"
  Product1/1 -> Add/1
  Subtract/1 -> Product1/1
  Compare To Constant/1 -> Logical Operator/1
  Bremse abschalten/1 -> Add/2
  v/1 -> Subtract/2, Compare To Constant/1, Compare To Constant1/1, Bremse abschalten/1, Subsystem/1(v)
  Gain/1 -> F_B,WB/1
  Product/1 -> Gain/1
  Constant2/1 -> Product/4
  Constant/1 -> Product/3
  Subsystem/1(y) -> Product/2
  Constant1/1 -> Subtract/1

== system NCS_Library/Controller/Logic/Braking Controller/konstante Fahrt/verfügbare Dynamische Bremskraft ==
  note: warum geteilt durch anzahl an angetriebenen wagen?
  v : Inport
  Add : Sum  Inputs=+++
  Add1 : Sum
  Compare To Constant : simulink/Logic and Bit Operations/Compare To Constant  relop=<=  const=29  OutDataTypeStr=boolean
  Compare To Constant1 : simulink/Logic and Bit Operations/Compare To Constant  relop=>  const=29  OutDataTypeStr=boolean
  Compare To Constant2 : simulink/Logic and Bit Operations/Compare To Constant  relop=>  const=4.2  OutDataTypeStr=boolean
  Compare To Constant3 : simulink/Logic and Bit Operations/Compare To Constant  relop=<=  const=4.2  OutDataTypeStr=boolean
  Compensate v=0 : Constant  Value=1e-10
  Divide : Product  Inputs=*/
  Fmax : Constant  Value=Fmaxdyn
  Fmax1 : Constant  Value=F_konst
  Gain : Gain  Gain=r_reib
  Gain1 : Gain  Gain=1/nW_an
  Leistung : Constant  Value=P_max
  Logical Operator : Logic  AllPortsSameDT=off  OutDataTypeStr=boolean
  Product : Product
  Product1 : Product
  Product2 : Product  Inputs=3
  Subtract : Sum  Inputs=+-
  F_B,dyn_max : Outport
  wires:
  Gain1/1 -> F_B,dyn_max/1
  Add1/1 -> Divide/2
  Product2/1 -> Add/1
  v/1 -> Compare To Constant1/1, Add1/1, Gain/1, Compare To Constant/1, Compare To Constant2/1, Product2/3, Compare To Constant3/1
  Fmax1/1 -> Product2/1
  Compare To Constant2/1 -> Logical Operator/2
  Logical Operator/1 -> Product/2
  Compensate v=0/1 -> Add1/2
  Compare To Constant1/1 -> Product1/2
  Add/1 -> Gain1/1
  Product1/1 -> Add/3
  Divide/1 -> Product1/1
  Product/1 -> Add/2
  Compare To Constant/1 -> Logical Operator/1
  Subtract/1 -> Product/1
  Gain/1 -> Subtract/2
  Fmax/1 -> Subtract/1
  Leistung/1 -> Divide/1
  Compare To Constant3/1 -> Product2/2

== system NCS_Library/Network/CAN/CAN Node 1/Signal To CAN Message/Set the Attributes of Messages ==
  InData : Inport
  initMessage : TriggerPort  TriggerType=function-call  IsSimulinkFunction=on  FunctionName=initMessage  FunctionVisibility=scoped  VariantControl=Variant
  CommDelay : Constant  Value=(49+8*MsgSize)/BUSCapacity  SampleTime=-1
  Constant : Constant  Value=SensorType  OutDataTypeStr=uint8
  Digital Clock : DigitalClock  SampleTime=-1
  ID : Constant  Value=MsgID  SampleTime=-1
  RTR : Constant  Value=0  SampleTime=-1
  Size : Constant  Value=MsgSize  SampleTime=-1
  ID~ : ArgOut  ArgumentName=ID
  RTR~ : ArgOut  Port=2  ArgumentName=RTR
  Size~ : ArgOut  Port=3  ArgumentName=Size
  Data : ArgOut  Port=4  ArgumentName=Data
  CommDelay~ : ArgOut  Port=5  ArgumentName=CommDelay
  Time : ArgOut  Port=6  ArgumentName=Time
  Type : ArgOut  Port=7  OutDataTypeStr=uint8  ArgumentName=Type
  wires:
  Constant/1 -> Type/1
  Digital Clock/1 -> Time/1
  Size/1 -> Size~/1
  RTR/1 -> RTR~/1
  ID/1 -> ID~/1
  CommDelay/1 -> CommDelay~/1
  InData/1 -> Data/1

== system NCS_Library/Network/CAN/CAN Node 2/Signal To CAN Message/Set the Attributes of Messages ==
  InData : Inport
  initMessage : TriggerPort  TriggerType=function-call  IsSimulinkFunction=on  FunctionName=initMessage  FunctionVisibility=scoped  VariantControl=Variant
  CommDelay : Constant  Value=(49+8*MsgSize)/BUSCapacity  SampleTime=-1
  Constant : Constant  Value=SensorType  OutDataTypeStr=uint8
  Digital Clock : DigitalClock  SampleTime=-1
  ID : Constant  Value=MsgID  SampleTime=-1
  RTR : Constant  Value=0  SampleTime=-1
  Size : Constant  Value=MsgSize  SampleTime=-1
  ID~ : ArgOut  ArgumentName=ID
  RTR~ : ArgOut  Port=2  ArgumentName=RTR
  Size~ : ArgOut  Port=3  ArgumentName=Size
  Data : ArgOut  Port=4  ArgumentName=Data
  CommDelay~ : ArgOut  Port=5  ArgumentName=CommDelay
  Time : ArgOut  Port=6  ArgumentName=Time
  Type : ArgOut  Port=7  OutDataTypeStr=uint8  ArgumentName=Type
  wires:
  InData/1 -> Data/1
  CommDelay/1 -> CommDelay~/1
  ID/1 -> ID~/1
  RTR/1 -> RTR~/1
  Size/1 -> Size~/1
  Digital Clock/1 -> Time/1
  Constant/1 -> Type/1

== system NCS_Library/Network/CAN/CAN Node 3/ACK Takt/Simulink Function3 ==
  Gate_ACK : TriggerPort  TriggerType=function-call  IsSimulinkFunction=on  FunctionName=Gate_ACK  FunctionVisibility=scoped  VariantControl=Variant
  Message Send : MessageSend  OutputPortMessageModes=m
      settings: InputPortMap=u1
  u : ArgIn  DisableCoverage=on  ArgumentName=u
  ctrl : Outport  InitialOutput=0
  wires:
  u/1 -> Message Send/1
  Message Send/1 -> ctrl/1

== system NCS_Library/Network/CAN/CAN Node 3/RX Takt/Simulink Function8 ==
  Gate_RX : TriggerPort  TriggerType=function-call  IsSimulinkFunction=on  FunctionName=Gate_RX  FunctionVisibility=scoped  VariantControl=Variant
  Message Send : MessageSend  OutputPortMessageModes=m
      settings: InputPortMap=u1
  u : ArgIn  DisableCoverage=on  ArgumentName=u
  ctrl : Outport  InitialOutput=0
  wires:
  Message Send/1 -> ctrl/1
  u/1 -> Message Send/1

== system NCS_Library/Network/CAN/CAN Node 4/ACK Takt/Simulink Function3 ==
  Gate_ACK : TriggerPort  TriggerType=function-call  IsSimulinkFunction=on  FunctionName=Gate_ACK  FunctionVisibility=scoped  VariantControl=Variant
  Message Send : MessageSend  OutputPortMessageModes=m
      settings: InputPortMap=u1
  u : ArgIn  DisableCoverage=on  ArgumentName=u
  ctrl : Outport  InitialOutput=0
  wires:
  Message Send/1 -> ctrl/1
  u/1 -> Message Send/1

== system NCS_Library/Network/CAN/CAN Node 4/RX Takt/Simulink Function8 ==
  Gate_RX : TriggerPort  TriggerType=function-call  IsSimulinkFunction=on  FunctionName=Gate_RX  FunctionVisibility=scoped  VariantControl=Variant
  Message Send : MessageSend  OutputPortMessageModes=m
      settings: InputPortMap=u1
  u : ArgIn  DisableCoverage=on  ArgumentName=u
  ctrl : Outport  InitialOutput=0
  wires:
  u/1 -> Message Send/1
  Message Send/1 -> ctrl/1

== system NCS_Library/Network/CAN/Logik/Fast_to_Slow/Measurement ==
  measure : Inport
  Detect Change2 : simulink/Logic and Bit Operations/Detect Change  vinit=0  OutDataTypeStr=boolean
  Digital Clock2 : DigitalClock  SampleTime=0.01
  Enabled Subsystem3 : Subsystem  TreatAsAtomicUnit=on
  Entity Terminator9 : EntityTerminator  InputPortMessageModes=m  EntryAction=getData(entity.Time);  NumberEntitiesArrived=on
      settings: OutputPortMap=o0
  Scope1 : Scope
  Scope4 : Scope
  Simulink Function7 : Subsystem  TreatAsAtomicUnit=on
  delay : Outport
  wires:
  Detect Change2/1 -> Enabled Subsystem3/Enable
  Simulink Function7/1(time) -> Enabled Subsystem3/2(time_sent), Scope4/1
  Entity Terminator9/1 -> Detect Change2/1, Scope1/1
  Digital Clock2/1 -> Enabled Subsystem3/1(time_arrived)
  Enabled Subsystem3/1(delay) -> delay/1
  measure/1 -> Entity Terminator9/1

== system NCS_Library/Network/CAN/Logik/Fast_to_Slow/Slow Takt ==
  In : Inport
  Entity Takt : EntityGenerator  OutputPortMessageModes=m  TimeSource=Signal port  Period=7  AttributeName=entity  EntityTypeName=gate  EntityPriority=1  DataInitialValue=1
      settings: InputPortMap=u1
  Entity Terminator13 : EntityTerminator  InputPortMessageModes=m
  Gate_5 : EntityGate  InputPortMessageModes=m,m  OutputPortMessageModes=m
  Offset [s] : Constant  Value=Offset
  Server : EntityServer  InputPortMessageModes=m  OutputPortMessageModes=m  Capacity=1  ServiceTimeValue=0  EntryAction=Gate_5(0);
  Server Offset : EntityServer  InputPortMessageModes=n,m  OutputPortMessageModes=m  Capacity=inf  ServiceTimeSource=Signal port  ServiceTimeValue=5
      settings: InputPortMap=u0,u2
  Server Takt : EntityServer  InputPortMessageModes=m  OutputPortMessageModes=m  Capacity=1  ServiceTimeValue=0.001  ServiceTimeAttributeName=CommDelay  EntryAction=Gate_5(1);  ExitAction=Gate_5(0);  SortingAttributeName=ID
  Simulink Function3 : Subsystem  TreatAsAtomicUnit=on
  Takt [s] : Constant  Value=Takt_slow
  Out : Outport
  wires:
  Server/1 -> Out/1
  Gate_5/1 -> Server/1
  In/1 -> Gate_5/2
  Simulink Function3/1(ctrl) -> Gate_5/1
  Entity Takt/1 -> Server Offset/2
  Server Offset/1 -> Server Takt/1
  Server Takt/1 -> Entity Terminator13/1
  Takt [s]/1 -> Entity Takt/1
  Offset [s]/1 -> Server Offset/1

== system NCS_Library/Network/CAN/Logik/Fast_to_Slow/Wait Takt ==
  In : Inport
  Entity Takt : EntityGenerator  OutputPortMessageModes=m  TimeSource=Signal port  Period=7  AttributeName=entity  EntityTypeName=gate  EntityPriority=10  DataInitialValue=1
      settings: InputPortMap=u1
  Entity Terminator13 : EntityTerminator  InputPortMessageModes=m
  Gate_4 : EntityGate  InputPortMessageModes=m,m  OutputPortMessageModes=m
  Offset [s] : Constant  Value=Offset
  Server ACK : EntityServer  InputPortMessageModes=m  OutputPortMessageModes=m  Capacity=1  ServiceTimeValue=0  EntryAction=Gate_4(Wait_off);
  Server Offset : EntityServer  InputPortMessageModes=n,m  OutputPortMessageModes=m  Capacity=inf  ServiceTimeSource=Signal port  ServiceTimeValue=5
      settings: InputPortMap=u0,u2
  Server Takt : EntityServer  InputPortMessageModes=m  OutputPortMessageModes=m  Capacity=1  ServiceTimeValue=0.001  ServiceTimeAttributeName=CommDelay  EntryAction=Gate_4(1);  ExitAction=Gate_4(Wait_off);  SortingAttributeName=ID
  Simulink Function3 : Subsystem  TreatAsAtomicUnit=on
  Takt [s] : Constant  Value=Takt_wait
  Out : Outport
  wires:
  Offset [s]/1 -> Server Offset/1
  Takt [s]/1 -> Entity Takt/1
  Server Takt/1 -> Entity Terminator13/1
  Server Offset/1 -> Server Takt/1
  Entity Takt/1 -> Server Offset/2
  Simulink Function3/1(ctrl) -> Gate_4/1
  In/1 -> Gate_4/2
  Gate_4/1 -> Server ACK/1
  Server ACK/1 -> Out/1

== system NCS_Library/Network/CAN/Logik/Slow_to_Fast/Copy Takt ==
  In : Inport
  Entity Replicator6 : EntityReplicator  InputPortMessageModes=m  OutputPortMessageModes=m,m
  Entity Takt : EntityGenerator  OutputPortMessageModes=m  TimeSource=Signal port  Period=7  AttributeName=entity  EntityTypeName=gate  EntityPriority=999  DataInitialValue=1
      settings: InputPortMap=u1
  Entity Terminator13 : EntityTerminator  InputPortMessageModes=m
  Entity Terminator3 : EntityTerminator  InputPortMessageModes=m  EntryAction=Gate_copy(0);  NumberEntitiesArrived=on
      settings: OutputPortMap=o0
  Gate_copy : EntityGate  InputPortMessageModes=m,m  OutputPortMessageModes=m
  Offset [s] : Constant  Value=Offset
  Scope4 : Scope
  Server Offset : EntityServer  InputPortMessageModes=n,m  OutputPortMessageModes=m  Capacity=inf  ServiceTimeSource=Signal port  ServiceTimeValue=5
      settings: InputPortMap=u0,u2
  Server Takt : EntityServer  InputPortMessageModes=m  OutputPortMessageModes=m  Capacity=1  ServiceTimeValue=0  ServiceTimeAttributeName=CommDelay  EntryAction=Gate_copy(1);  ExitAction=Gate_copy(0);  SortingAttributeName=ID
  Simulink Function3 : Subsystem  TreatAsAtomicUnit=on
  Takt_fast [s] : Constant  Value=Takt_fast
  Out : Outport
  wires:
  Entity Replicator6/2 -> Out/1
  Entity Replicator6/1 -> Entity Terminator3/1
  Entity Terminator3/1 -> Scope4/1
  Offset [s]/1 -> Server Offset/1
  Takt_fast [s]/1 -> Entity Takt/1
  Server Takt/1 -> Entity Terminator13/1
  Server Offset/1 -> Server Takt/1
  Entity Takt/1 -> Server Offset/2
  Simulink Function3/1(ctrl) -> Gate_copy/1
  In/1 -> Gate_copy/2
  Gate_copy/1 -> Entity Replicator6/1

== system NCS_Library/Network/CAN/Logik/Slow_to_Fast/Fast Takt ==
  In : Inport
  Entity Takt : EntityGenerator  OutputPortMessageModes=m  TimeSource=Signal port  Period=7  AttributeName=entity  EntityTypeName=gate  EntityPriority=1  DataInitialValue=1
      settings: InputPortMap=u1
  Entity Terminator13 : EntityTerminator  InputPortMessageModes=m
  Gate : EntityGate  InputPortMessageModes=m,m  OutputPortMessageModes=m
  Offset [s] : Constant  Value=Offset
  Server : EntityServer  InputPortMessageModes=m  OutputPortMessageModes=m  Capacity=1  ServiceTimeValue=0  EntryAction=Gate(0);
  Server Offset : EntityServer  InputPortMessageModes=n,m  OutputPortMessageModes=m  Capacity=inf  ServiceTimeSource=Signal port  ServiceTimeValue=5
      settings: InputPortMap=u0,u2
  Server Takt : EntityServer  InputPortMessageModes=m  OutputPortMessageModes=m  Capacity=1  ServiceTimeValue=0.001  ServiceTimeAttributeName=CommDelay  EntryAction=Gate(1);  ExitAction=Gate(0);  SortingAttributeName=ID
  Simulink Function3 : Subsystem  TreatAsAtomicUnit=on
  Takt_fast [s] : Constant  Value=Takt_fast
  Out : Outport
  wires:
  Offset [s]/1 -> Server Offset/1
  Takt_fast [s]/1 -> Entity Takt/1
  Server Takt/1 -> Entity Terminator13/1
  Server Offset/1 -> Server Takt/1
  Entity Takt/1 -> Server Offset/2
  Simulink Function3/1(ctrl) -> Gate/1
  In/1 -> Gate/2
  Gate/1 -> Server/1
  Server/1 -> Out/1
